simulink model "DC_MOTOR_2014a"  (R2014a)
settings: Solver=ode45  SolverMode=SingleTasking  StartTime=0.0  StopTime=10.0  RelTol=1e-3
values from neighbouring files (symbols this model uses):
  J = 0.02    [DC_parameters.m]
  Kemf = 0.1    [DC_parameters.m]
  Kf = 0.2    [DC_parameters.m]
  Km = 0.1    [DC_parameters.m]
  L = 0.5    [DC_parameters.m]
  R = 2    [DC_parameters.m]
settings Model: CovMetricSettings=dwe  CovHtmlReporting=off  covSaveCumulativeToWorkspaceVar=off  CovSaveSingleToWorkspaceVar=off  CovExternalEMLEnable=on  CovSFcnEnable=on  Creator=wangyue  LastModifiedBy=wangyue
settings DataIOCC: LimitDataPoints=off  SaveFormat=StructureWithTime  ReturnWorkspaceOutputs=on
settings DebuggingCC: MergeDetectMultiDrivingBlocksExec=error  SolverPrmCheckMsg=none  FrameProcessingCompatibilityMsg=error  SFUnexpectedBacktrackingDiag=error  SFNoUnconditionalDefaultTransitionDiag=error
settings HardwareCC: ProdBitPerPointer=64  ProdLargestAtomicFloat=Float  ProdIntDivRoundTo=Zero  ProdEndianess=LittleEndian  ProdHWDeviceType=Specified
settings ModelReferenceCC: PropagateSignalLabelsOutOfModel=on
settings SFSimCC: SimUseLocalCustomCode=on
settings RTWCC: RTWUseLocalCustomCode=on
settings GRTTargetCC: TargetLangStandard=C99 (ISO)

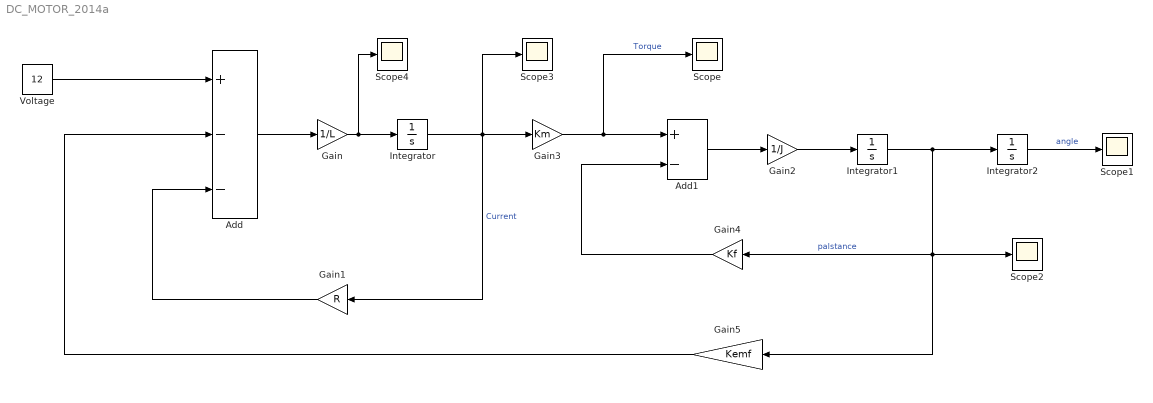
== system DC_MOTOR_2014a ==
  Add : Sum  Inputs=+--
  Add1 : Sum  Inputs=+-
  Gain : Gain  Gain=1/L
  Gain1 : Gain  Gain=R
  Gain2 : Gain  Gain=1/J
  Gain3 : Gain  Gain=Km
  Gain4 : Gain  Gain=Kf
  Gain5 : Gain  Gain=Kemf
  Integrator : Integrator
  Integrator1 : Integrator
  Integrator2 : Integrator
  Scope{,1..4} (5 alike) : Scope
      Scope settings: TimeRange=auto  MaxDataPoints=5000  SaveToWorkspace=off  SaveName=ScopeData  YMin=-0.07317  YMax=0.65854  SampleTime=-1
      Scope1 settings: TimeRange=auto  MaxDataPoints=5000  SaveToWorkspace=off  YMin=-3.53361  YMax=31.8025  SampleTime=-1
      Scope2 settings: TimeRange=auto  MaxDataPoints=5000  SaveToWorkspace=off  SaveName=ScopeData2  YMin=-0.36585  YMax=3.29268  SampleTime=-1
      Scope3 settings: TimeRange=auto  MaxDataPoints=5000  SaveToWorkspace=off  SaveName=ScopeData3  YMin=-0.73171  YMax=6.58537  SampleTime=-1
      Scope4 settings: TimeRange=auto  MaxDataPoints=5000  SaveToWorkspace=off  SaveName=ScopeData4  YMin=-3.00000  YMax=27.00000  SampleTime=-1
  Voltage : Constant  Value=12
  wires:
  Add/1 -> Gain/1
  Voltage/1 -> Add/1
  Gain/1 -> Scope4/1, Integrator/1
  Integrator/1 -> Scope3/1, Gain3/1, Gain1/1  "Current"
  Add1/1 -> Gain2/1
  Gain3/1 -> Scope/1, Add1/1  "Torque"
  Gain2/1 -> Integrator1/1
  Integrator1/1 -> Integrator2/1, Scope2/1, Gain4/1, Gain5/1  "palstance"
  Gain4/1 -> Add1/2
  Gain1/1 -> Add/3
  Gain5/1 -> Add/2
  Integrator2/1 -> Scope1/1  "angle"
